simulink model "abslut125_fixpt16"  (R2021b)
settings: Solver=VariableStepAuto  StartTime=0.0  StopTime=359  RelTol=1e-3
undefined symbols (not defined in the file or in its folder): S, vsva2197, xcvc1902
libraries: hdlBasic x1350, vmcUtilities x1
(part 1 of 8)
settings Model: Creator=shu_abe  LastModifiedBy=shu_abe

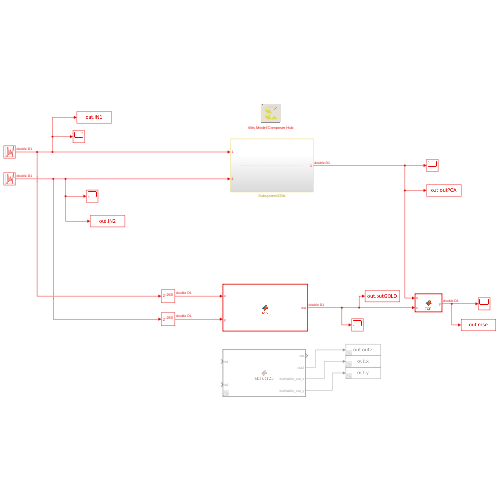
[thumbnail: Simulink's stored preview of the top-level diagram]
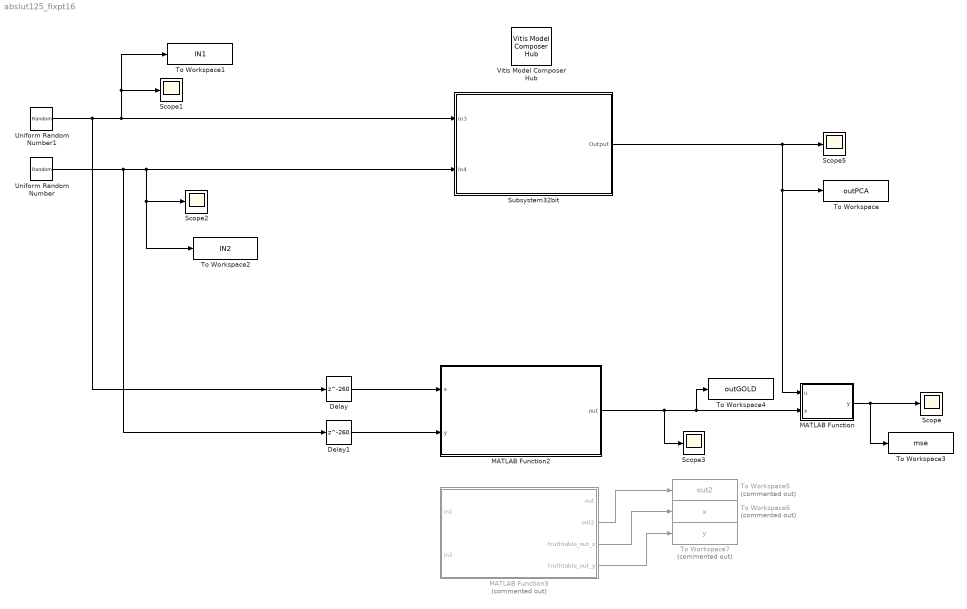
== system abslut125_fixpt16 ==
  Delay : Delay  DelayLength=260
  Delay1 : Delay  DelayLength=260
  MATLAB Function : MATLAB Function  TreatAsAtomicUnit=on
  MATLAB Function2 : MATLAB Function  TreatAsAtomicUnit=on
  MATLAB Function3 : MATLAB Function  Commented=on  TreatAsAtomicUnit=on
  Scope{,1..3,5} (5 alike) : Scope
  Subsystem32bit : Subsystem
  To Workspace : ToWorkspace  VariableName=outPCA  SaveFormat=Structure With Time  SampleTime=1
  To Workspace1 : ToWorkspace  VariableName=IN1  SaveFormat=Structure With Time  SampleTime=-1
  To Workspace2 : ToWorkspace  VariableName=IN2  SaveFormat=Structure With Time  SampleTime=-1
  To Workspace3 : ToWorkspace  VariableName=mse  SaveFormat=Structure With Time  SampleTime=1
  To Workspace4 : ToWorkspace  VariableName=outGOLD  SaveFormat=Structure With Time  SampleTime=1
  To Workspace5 : ToWorkspace  Commented=on  VariableName=out2  SaveFormat=Structure With Time  SampleTime=1
  To Workspace6 : ToWorkspace  Commented=on  VariableName=x  SaveFormat=Structure With Time  SampleTime=1
  To Workspace7 : ToWorkspace  Commented=on  VariableName=y  SaveFormat=Structure With Time  SampleTime=1
  Uniform Random Number : UniformRandomNumber  SampleTime=1
  Uniform Random Number1 : UniformRandomNumber  Seed=1  SampleTime=1
  Vitis Model Composer Hub : vmcUtilities/Vitis Model Composer Hub  Tag=genX  CodeGeneration=off  SubsystemName=<enter or select subsystem name>  TargetDirectory=./code  ExportType=HLS C++ code  IpVendor=xilinx.com  IpLibrary=hls  IpVersion=1.0  IpHWLanguage=Verilog  AieCompilerOptions={}  CreateTestbench=off  TestbenchStackSize=10  RunAieSim=off  AieSimTimeout=50000  RunAieSimProfiling=off  LaunchVitisAnalyzer=off  PlotOutput=off  RunX86Sim=off  X86SimTimeout=10  GenHwImage=off  PlatformType=Not Specified  HwSystemType=Baremetal  HwValidationTarget=hw  ProjDevice=Alveo U250 Data Center Accelerator Card (xcu250-figd2104-2L-e)  ProjDevicePart=xcvc1902-vsva2197-2MP-e-S  SamplePeriod=-1  ClockFrequency=200  DataPathParallelism=1  xilinxfamily=virtexuplus  part=xcu250  speed=-2L-e  package=figd2104  directory=./abslut125_fixpt32  testbench=off  incr_netlist=off  synthesis_tool=Vivado  clock_wrapper=Clock Enables  dbl_ovrd=According to Block Masks  dcm_input_clock_period=10  sysclk_period=50  simulink_period=1  eval_field=0
  wires:
  MATLAB Function/1(y) -> Scope/1, To Workspace3/1
  Subsystem32bit/1(Output) -> Scope5/1, MATLAB Function/1(u), To Workspace/1
  Uniform Random Number1/1 -> Subsystem32bit/1(In3), To Workspace1/1, Scope1/1, Delay/1
  Uniform Random Number/1 -> Subsystem32bit/2(In4), To Workspace2/1, Scope2/1, Delay1/1
  MATLAB Function2/1(out) -> Scope3/1, To Workspace4/1, MATLAB Function/2(x)
  Delay/1 -> MATLAB Function2/1(x)
  Delay1/1 -> MATLAB Function2/2(y)
  MATLAB Function3/2(out2) -> To Workspace5/1
  MATLAB Function3/3(truthtable_out_x) -> To Workspace6/1
  MATLAB Function3/4(truthtable_out_y) -> To Workspace7/1
